simulink model "Red_problema7_imc_v2021"  (R2021a)
settings: Solver=ode15s  StartTime=0.0  StopTime=sim_time  RelTol=1e-3
values from neighbouring files (symbols this model uses):
  aE1 = a121_f    (= 50.6984417257)    [inicializar_areas_ej7.m]
  aE2 = a112_f    (= 77.7288481128)    [inicializar_areas_ej7.m]
  aE3 = a222_f    (= 163.424628674)    [inicializar_areas_ej7.m]
  aE4 = a213_f    (= 304.960661681)    [inicializar_areas_ej7.m]
  aEcu1 = aEcu1_f    (= 4.92677788377)    [inicializar_areas_ej7.m]
  aEcu2 = aEcu2_f    (= 18.7854640224)    [inicializar_areas_ej7.m]
  aEhu2 = aEhu2_f    (= 81.1441370104)    [inicializar_areas_ej7.m]
  d1_end = 0    [script_build_tfs.m]    (also in todo_nom_full.m; todo_nom_spar.m)
  d1_in = 0    [script_build_tfs.m]    (also in todo_nom_full.m; todo_nom_spar.m)
  d2_end = 0    [script_build_tfs.m]    (also in todo_nom_full.m; todo_nom_spar.m)
  d2_in = 0    [script_build_tfs.m]    (also in todo_nom_full.m; todo_nom_spar.m)
  d3_end = 0    [script_build_tfs.m]    (also in todo_nom_full.m; todo_nom_spar.m)
  d3_in = 0    [script_build_tfs.m]    (also in todo_nom_full.m; todo_nom_spar.m)
  d4_end = 0    [script_build_tfs.m]    (also in todo_nom_full.m; todo_nom_spar.m)
  d4_in = 0    [script_build_tfs.m]    (also in todo_nom_full.m; todo_nom_spar.m)
  d5_end = 0    [script_build_tfs.m]    (also in todo_nom_full.m; todo_nom_spar.m)
  d5_in = 0    [script_build_tfs.m]    (also in todo_nom_full.m; todo_nom_spar.m)
  d6_end = 0    [script_build_tfs.m]    (also in todo_nom_full.m; todo_nom_spar.m)
  d6_in = 0    [script_build_tfs.m]    (also in todo_nom_full.m; todo_nom_spar.m)
  d7_end = 0    [script_build_tfs.m]    (also in todo_nom_full.m; todo_nom_spar.m)
  d7_in = 0    [script_build_tfs.m]    (also in todo_nom_full.m; todo_nom_spar.m)
  d8_end = 0    [script_build_tfs.m]    (also in todo_nom_full.m; todo_nom_spar.m)
  d8_in = 0    [script_build_tfs.m]    (also in todo_nom_full.m; todo_nom_spar.m)
  fcu2 = 5    [ini_comun.m]    (also in inicializar_areas_ej7.m; script_build_tfs.m; script_ini_ej7.m)
  fhu2 = 15    [ini_comun.m]    (also in inicializar_areas_ej7.m; script_build_tfs.m; script_ini_ej7.m)
  hcu = 1    [ini_comun.m]    (also in script_build_tfs.m; script_ini_ej7.m)
  hhu = 1    [ini_comun.m]    (also in script_build_tfs.m; script_ini_ej7.m)
  initials = nominales_u_full    [script_build_tfs.m]    (also in script_desc.m = nominales_u_desc; script_full.m; script_ini_ej7.m; script_spar.m = nominales_u_spar)
  s1 = 30    [ini_comun.m]    (also in script_build_tfs.m; script_ini_ej7.m)
  salida_pto_op = [432.98548652 333.041991092 482.910853128 483.037830645]    [D_desc_v1.mat]    (also in D_full_v1.mat = [432.959604691 333.033592475 482.878829311 483.126301479]; D_spar_v1.mat = [433.148784168 333.052277913 483.093095371 482.96198908]; salida_pt_op_desc.mat = [432.94450339 332.966292174 482.988443985 483.057252903]; salida_pt_op_desc_v2021.mat)
  setpoints = [160+273 60+273 210+273 210+273]    [ini_comun.m]    (also in script_build_tfs.m; script_ini_ej7.m)
  switch_var = 2    [script_IMC_ej7.m]    (also in script_desc.m = 0; script_full.m; script_spar.m = 1)
  t_step = 2000    [ini_comun.m]    (also in script_build_tfs.m = 300; script_ini_ej7.m = 600; validacion.m = 500)
  Tcuin = 288    [ini_comun.m]    (also in script_build_tfs.m; script_ini_ej7.m)
  Thuin = 523    [ini_comun.m]    (also in script_build_tfs.m; script_ini_ej7.m)
libraries: simulink x5, cstblocks x2
(part 1 of 2)
settings Model: Creator=Lautaro  LastModifiedBy=fzpat
settings SolverCC: AlgebraicLoopSolver=TrustRegion
settings DataIOCC: LimitDataPoints=on  SaveFormat=Array  ReturnWorkspaceOutputs=off
settings OptimizationCC: BlockReduction=off  BooleanDataType=off  LifeSpan=inf
settings DebuggingCC: SaveWithParameterizedLinksMsg=none  UnderspecifiedInitializationDetection=Classic  MergeDetectMultiDrivingBlocksExec=none  SignalResolutionControl=TryResolveAllWithWarning  SFUnexpectedBacktrackingDiag=warning  SFNoUnconditionalDefaultTransitionDiag=warning  SFExecutionAtInitializationDiag=none  ArithmeticOperatorsInVariantConditions=warning
settings HardwareCC: ProdBitPerPointer=32  ProdBitPerSizeT=32  ProdBitPerPtrDiffT=32  ProdLargestAtomicFloat=None  ProdIntDivRoundTo=Undefined  ProdEndianess=Unspecified  ProdWordSize=32  ProdHWDeviceType=32-bit Generic  TargetUnknown=on
settings ModelReferenceCC: PropagateSignalLabelsOutOfModel=off
settings SFSimCC: SimUseLocalCustomCode=off  CustomCodeUndefinedFunction=UseInterfaceOnly
settings RTWCC: RTWUseLocalCustomCode=off
settings CodeAppCC: StateflowObjectComments=on
settings GRTTargetCC: TargetLangStandard=C89/C90 (ANSI)
settings ConfigComp: CovMetricSettings=dw  CovSaveCumulativeToWorkspaceVar=on  CovSaveSingleToWorkspaceVar=on  CovExternalEMLEnable=off  CovSFcnEnable=off

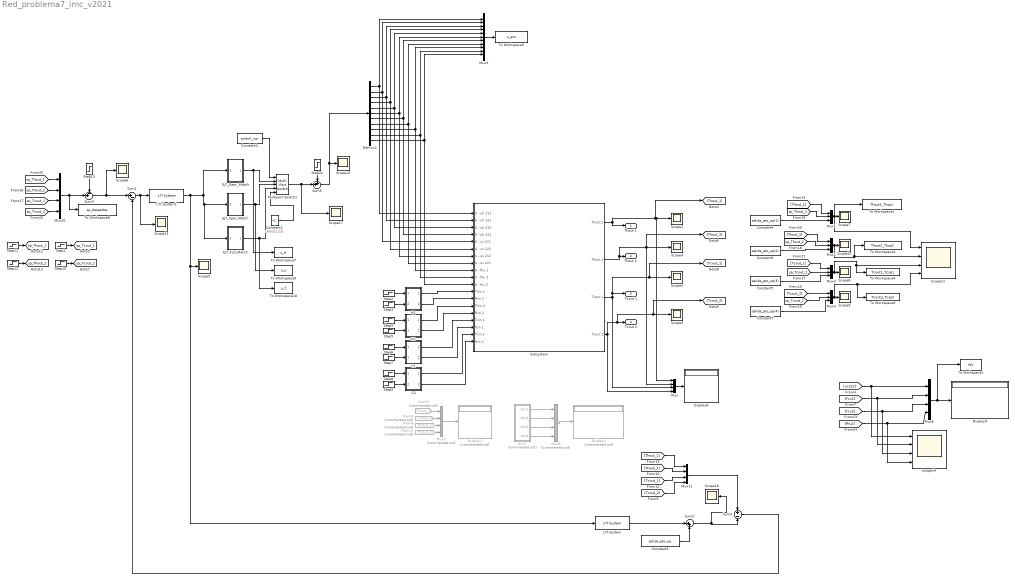
== system Red_problema7_imc_v2021 ==
  C1 : Subsystem
  "C2 " : Subsystem
  Constant1 : Constant  Value=zeros(1,11)
  Constant2 : Constant  Value=switch_var
  Constant3 : Constant  Value=salida_pto_op
  Constant4 : Constant  Value=salida_pto_op(1)
  Constant5 : Constant  Value=salida_pto_op(3)
  Constant6 : Constant  Value=salida_pto_op(2)
  Constant7 : Constant  Value=salida_pto_op(4)
  Demux2 : Demux  Outputs=11
  Display1 : Display  Commented=on
  Display5 : Display  Commented=on
  Display8 : Display
  Display9 : Display
  Ej7_Desc_Match : Subsystem
  Ej7_Full_Match : Subsystem
  Ej7_Spar_Match : Subsystem
  From11 : From  Commented=on  GotoTag=Tcout_2  TagVisibility=global
  From5 : From  Commented=on  GotoTag=Thout_1  TagVisibility=global
  From6 : From  Commented=on  GotoTag=Thout_2  TagVisibility=global
  From8 : From  Commented=on  GotoTag=Tcout_1  TagVisibility=global
  "H1 " : Subsystem
  H2 : Subsystem
  LTI System : cstblocks/LTI System  sys=Gimc  IC=[]
  LTI System1 : cstblocks/LTI System  sys=Kimc_u  IC=[]
  Multiport Switch1 : MultiPortSwitch  DataPortOrder=Zero-based contiguous  DataPortForDefault=Additional data port  DiagnosticForDefault=None  zeroidx=on
  Mux{,6,10..11} (4 alike) : Mux
  Mux{1..4} (4 alike) : Mux  Inputs=3
  Mux5 : Mux  Inputs=11
  Mux7 : Mux  Commented=on
  Mux8 : Mux  Commented=on
  Scope{1..10,12..13,17..18} (14 alike) : Scope
  Scope11 : Scope  NumInputPorts=4
  Scope14 : Scope  NumInputPorts=4
  Step1 : Step  Time=1e9  Before=210+273  After=210+273
  Step10 : Step  Time=1e10  Before=210+273  After=210+273
  Step11 : Step  Time=1e9  Before=160+273  After=160+273
  Step12 : Step  Time=1e9  Before=60+273  After=60+273
  Step13 : Step  Time=0  Before=setpoints  After=salida_pto_op
  Step2 : Step  Time=t_step  Before=d1_in  After=d1_end
  Step22 : Step  Time=0  Before=initials  After=initials
  Step3 : Step  Time=t_step  Before=d2_in  After=d2_end
  Step4 : Step  Time=t_step  Before=d3_in  After=d3_end
  Step5 : Step  Time=t_step  Before=d4_in  After=d4_end
  Step6 : Step  Time=t_step  Before=d5_in  After=d5_end
  Step7 : Step  Time=t_step  Before=d6_in  After=d6_end
  Step8 : Step  Time=t_step  Before=d7_in  After=d7_end
  Step9 : Step  Time=t_step  Before=d8_in  After=d8_end
  Subsystem : Subsystem
  Sum1 : Sum  Inputs=|+-
  Sum2 : Sum  Inputs=|++
  Sum3 : Sum  Inputs=+-
  Sum4 : Sum  Inputs=-+|
  Sum5 : Sum  Inputs=++|
  To Workspace1 : ToWorkspace  VariableName=MV  SaveFormat=Timeseries  SampleTime=-1
  To Workspace10 : ToWorkspace  VariableName=u_f  SaveFormat=Timeseries  SampleTime=-1
      settings: Save2DSignal=2-D array (concatenate along first dimension)
  To Workspace2 : ToWorkspace  VariableName=Thout1_Thsp1  SaveFormat=Timeseries  SampleTime=-1
  To Workspace3 : ToWorkspace  VariableName=Thout2_Thsp2  SampleTime=-1
  To Workspace4 : ToWorkspace  VariableName=Tcout1_Tcsp1  SampleTime=-1
  To Workspace5 : ToWorkspace  VariableName=u_exc  SaveFormat=Timeseries  SampleTime=-1
      settings: Save2DSignal=2-D array (concatenate along first dimension)
  To Workspace6 : ToWorkspace  VariableName=Tcout2_Tcsp2  SampleTime=-1
  To Workspace7 : ToWorkspace  VariableName=u_d  SaveFormat=Timeseries  SampleTime=-1
      settings: Save2DSignal=2-D array (concatenate along first dimension)
  To Workspace8 : ToWorkspace  VariableName=sp_deseados  SampleTime=-1
  To Workspace9 : ToWorkspace  VariableName=u_s  SaveFormat=Timeseries  SampleTime=-1
      settings: Save2DSignal=2-D array (concatenate along first dimension)
  error : Subsystem  Commented=on
  Thout 1 : Outport  VectorParamsAs1DForOutWhenUnconnected=off
  Thout 2 : Outport  Port=2  VectorParamsAs1DForOutWhenUnconnected=off
  Tcout 1 : Outport  Port=3  VectorParamsAs1DForOutWhenUnconnected=off
  Tcout 2 : Outport  Port=4  VectorParamsAs1DForOutWhenUnconnected=off
  tag scope: sp_Tcout_1=global, sp_Tcout_2=global, sp_Thout_1=global, sp_Thout_2=global
  wires:
  Subsystem/1(Thout 1) -> Thout 1/1, [Thout_1], Mux/1, Scope1/1
  Mux/1 -> Display8/1
  "H1 "/1(Out1) -> Subsystem/12(Thin 1)
  "H1 "/2(Out2) -> Subsystem/13(fhin 1)
  H2/2(Out2) -> Subsystem/15(fhin 2)
  H2/1(Out1) -> Subsystem/14(Thin 2)
  C1/1(Out1) -> Subsystem/16(Tcin 1)
  C1/2(Out2) -> Subsystem/17(fcin 1)
  "C2 "/1(Out1) -> Subsystem/18(Tcin 2)
  "C2 "/2(Out2) -> Subsystem/19(fcin 2)
  Subsystem/2(Thout 2) -> [Thout_2], Scope4/1, Mux/2, Thout 2/1
  Subsystem/3(Tcout 1) -> [Tcout_1], Scope2/1, Tcout 1/1, Mux/3
  Step2/1 -> "H1 "/1(Thin 1)
  Step3/1 -> "H1 "/2(fhin 1)
  Step4/1 -> H2/1(Thin 1)
  Step5/1 -> H2/2(fhin 1)
  Step6/1 -> C1/1(Tcin 1)
  Step7/1 -> C1/2(fcin 1)
  Step8/1 -> "C2 "/1(Tcin 2)
  Step9/1 -> "C2 "/2(fcin 2)
  Subsystem/4(Tcout 2) -> [Tcout_2], Scope3/1, Tcout 2/1, Mux/4
  Mux5/1 -> To Workspace5/1
  Mux7/1 -> Display1/1
  From6/1 -> Mux7/2
  error/3(Out3) -> Mux8/3
  From5/1 -> Mux7/1
  From11/1 -> Mux7/4
  From8/1 -> Mux7/3
  error/4(Out4) -> Mux8/4
  Mux8/1 -> Display5/1
  Step12/1 -> [sp_Thout_2]
  Step11/1 -> [sp_Thout_1]
  Step1/1 -> [sp_Tcout_1]
  Step10/1 -> [sp_Tcout_2]
  error/2(Out2) -> Mux8/2
  error/1(Out1) -> Mux8/1
  [Tcout_1] -> Mux3/1
  Mux3/1 -> To Workspace4/1, Scope11/3, Scope8/1
  [Thout_2] -> Mux2/1
  [sp_Tcout_1] -> Mux3/2
  Mux1/1 -> To Workspace2/1, Scope11/1, Scope7/1
  Mux2/1 -> To Workspace3/1, Scope11/2, Scope10/1
  [Tcout_2] -> Mux4/1
  [Thout_1] -> Mux1/1
  Mux4/1 -> To Workspace6/1, Scope11/4, Scope9/1
  [sp_Thout_2] -> Mux2/2
  [sp_Tcout_2] -> Mux4/2
  [sp_Thout_1] -> Mux1/2
  [fcu1] -> Mux6/2, Scope14/2
  [fhu2] -> Scope14/4, Mux6/4
  [uc222] -> Mux6/1, Scope14/1
  [fcu2] -> Mux6/3, Scope14/3
  Mux6/1 -> To Workspace1/1, Display9/1
  [sp_Tcout_1] -> Mux10/3
  [sp_Thout_2] -> Mux10/2
  [sp_Thout_1] -> Mux10/1
  Sum2/1 -> Sum3/2, Scope18/1
  [sp_Tcout_2] -> Mux10/4
  Mux10/1 -> To Workspace8/1, Sum4/2
  Sum1/1 -> Scope13/1, LTI System1/1
  Ej7_Spar_Match/1(Out1) -> To Workspace9/1, Multiport Switch1/3
  Constant1/1 -> Multiport Switch1/5
  Ej7_Full_Match/1(Out1) -> To Workspace10/1, Multiport Switch1/4
  Ej7_Desc_Match/1(Out1) -> Multiport Switch1/2, To Workspace7/1
  Constant2/1 -> Multiport Switch1/1
  Mux11/1 -> Sum3/1
  [Thout_2] -> Mux11/2
  Constant3/1 -> Sum2/2
  [Tcout_1] -> Mux11/3
  [Thout_1] -> Mux11/1
  LTI System/1 -> Sum2/1
  [Tcout_2] -> Mux11/4
  Demux2/10 -> Subsystem/10(U - fhu 2), Mux5/10
  Step22/1 -> Sum5/1
  Demux2/4 -> Mux5/4, Subsystem/6(U - uc 121)
  Demux2/3 -> Mux5/3, Subsystem/2(U - uh 121)
  Demux2/7 -> Mux5/7, Subsystem/4(U - uh 221)
  Demux2/8 -> Mux5/8, Subsystem/8(U - uc 221)
  Demux2/11 -> Mux5/11, Subsystem/11(U - fcu 2)
  Demux2/5 -> Mux5/5, Subsystem/3(U - uh 212)
  Demux2/9 -> Subsystem/9(U - fhu 1), Mux5/9
  Demux2/6 -> Mux5/6, Subsystem/7(U - uc 212)
  Demux2/1 -> Mux5/1, Subsystem/1(U - uh 111)
  Demux2/2 -> Mux5/2, Subsystem/5(U - uc 111)
  Multiport Switch1/1 -> Scope17/1, Sum5/2
  Sum3/1 -> Sum1/2
  Sum4/1 -> Scope6/1, Sum1/1
  Step13/1 -> Sum4/1
  Sum5/1 -> Demux2/1, Scope12/1
  LTI System1/1 -> LTI System/1, Scope5/1, Ej7_Desc_Match/1(In1), Ej7_Full_Match/1(In1), Ej7_Spar_Match/1(In1)
  Constant4/1 -> Mux1/3
  Constant6/1 -> Mux2/3
  Constant5/1 -> Mux3/3
  Constant7/1 -> Mux4/3

== system Red_problema7_imc_v2021/C1 ==
  Tcin 1 : Inport
  fcin 1 : Inport  Port=2
  Add2 : Sum
  Add3 : Sum
  Constant3 : Constant  Value=50+273
  Constant4 : Constant  Value=20
  Out1 : Outport  VectorParamsAs1DForOutWhenUnconnected=off
  Out2 : Outport  Port=2  VectorParamsAs1DForOutWhenUnconnected=off
  wires:
  Constant3/1 -> Add2/1
  Constant4/1 -> Add3/1
  Tcin 1/1 -> Add2/2
  fcin 1/1 -> Add3/2
  Add2/1 -> Out1/1
  Add3/1 -> Out2/1

== system Red_problema7_imc_v2021/C2  ==
  Tcin 2 : Inport
  fcin 2 : Inport  Port=2
  Add4 : Sum
  Add5 : Sum
  Constant5 : Constant  Value=160+273
  Constant6 : Constant  Value=50
  Out1 : Outport  VectorParamsAs1DForOutWhenUnconnected=off
  Out2 : Outport  Port=2  VectorParamsAs1DForOutWhenUnconnected=off
  wires:
  Constant5/1 -> Add4/1
  Constant6/1 -> Add5/1
  Tcin 2/1 -> Add4/2
  fcin 2/1 -> Add5/2
  Add4/1 -> Out1/1
  Add5/1 -> Out2/1

== system Red_problema7_imc_v2021/Ej7_Desc_Match ==
  In1 : Inport
  Constant1 : Constant  Value=0
  Demux3 : Demux
  Mux10 : Mux  Inputs=11
  Out1 : Outport
  wires:
  In1/1 -> Demux3/1
  Constant1/1 -> Mux10/3, Mux10/5, Mux10/7, Mux10/6, Mux10/4, Mux10/2, Mux10/1
  Demux3/4 -> Mux10/11
  Demux3/2 -> Mux10/10
  Demux3/1 -> Mux10/9
  Mux10/1 -> Out1/1
  Demux3/3 -> Mux10/8

== system Red_problema7_imc_v2021/Ej7_Full_Match ==
  In1 : Inport
  Constant1 : Constant  Value=0
  Constant2 : Constant  Value=0
  Constant3 : Constant  Value=0
  Demux3 : Demux
  Mux10 : Mux  Inputs=11
  Out1 : Outport
  wires:
  Constant3/1 -> Mux10/11
  In1/1 -> Demux3/1
  Constant2/1 -> Mux10/7, Mux10/4, Mux10/3, Mux10/5, Mux10/6
  Constant1/1 -> Mux10/1
  Demux3/4 -> Mux10/8
  Demux3/3 -> Mux10/2
  Demux3/2 -> Mux10/10
  Demux3/1 -> Mux10/9
  Mux10/1 -> Out1/1

== system Red_problema7_imc_v2021/Ej7_Spar_Match ==
  In1 : Inport
  Constant1 : Constant  Value=0
  Constant2 : Constant  Value=0
  Demux3 : Demux
  Mux10 : Mux  Inputs=11
  Out1 : Outport
  wires:
  Mux10/1 -> Out1/1
  Demux3/1 -> Mux10/9
  Demux3/2 -> Mux10/10
  Demux3/3 -> Mux10/5
  Demux3/4 -> Mux10/11
  Constant1/1 -> Mux10/4, Mux10/3, Mux10/2, Mux10/1
  Constant2/1 -> Mux10/6, Mux10/8, Mux10/7
  In1/1 -> Demux3/1

== system Red_problema7_imc_v2021/H1  ==
  Thin 1 : Inport
  fhin 1 : Inport  Port=2
  Add : Sum
  Add1 : Sum
  Constant1 : Constant  Value=270+273
  Constant2 : Constant  Value=18
  Out1 : Outport  VectorParamsAs1DForOutWhenUnconnected=off
  Out2 : Outport  Port=2  VectorParamsAs1DForOutWhenUnconnected=off
  wires:
  Constant1/1 -> Add/1
  Thin 1/1 -> Add/2
  Add/1 -> Out1/1
  Constant2/1 -> Add1/1
  fhin 1/1 -> Add1/2
  Add1/1 -> Out2/1

== system Red_problema7_imc_v2021/H2 ==
  Thin 1 : Inport
  fhin 1 : Inport  Port=2
  Add : Sum
  Add1 : Sum
  Constant1 : Constant  Value=220+273
  Constant2 : Constant  Value=22
  Out1 : Outport  VectorParamsAs1DForOutWhenUnconnected=off
  Out2 : Outport  Port=2  VectorParamsAs1DForOutWhenUnconnected=off
  wires:
  Constant1/1 -> Add/1
  Thin 1/1 -> Add/2
  Add/1 -> Out1/1
  Constant2/1 -> Add1/1
  fhin 1/1 -> Add1/2
  Add1/1 -> Out2/1

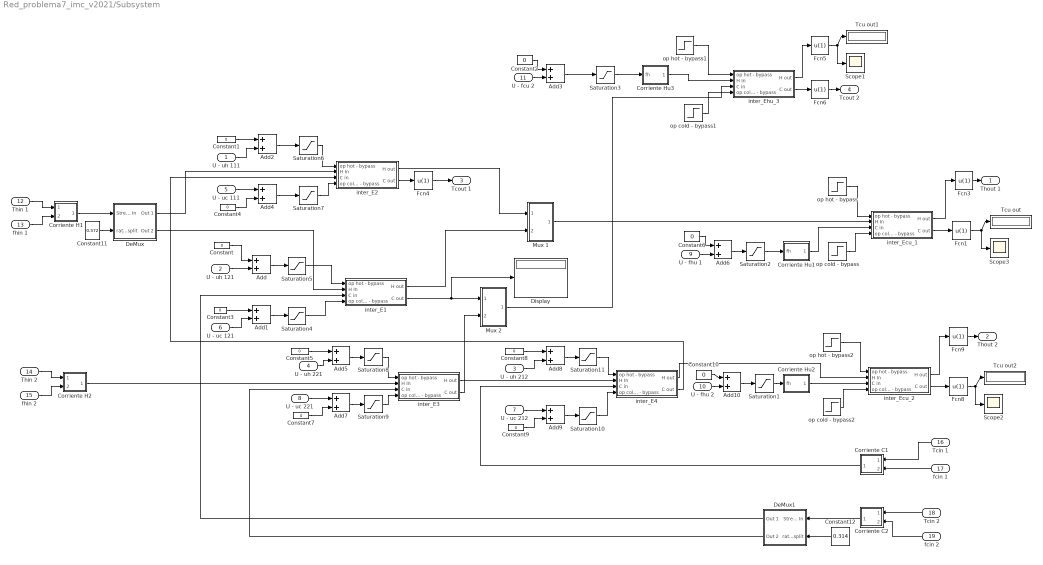
== system Red_problema7_imc_v2021/Subsystem ==
  U - uh 111 : Inport
  U - uh 121 : Inport  Port=2
  U - uh 212 : Inport  Port=3
  U - uh 221 : Inport  Port=4
  U - uc 111 : Inport  Port=5
  U - uc 121 : Inport  Port=6
  U - uc 212 : Inport  Port=7
  U - uc 221 : Inport  Port=8
  U - fhu 1 : Inport  Port=9
  U - fhu 2 : Inport  Port=10
  U - fcu 2 : Inport  Port=11
  Thin 1 : Inport  Port=12
  fhin 1 : Inport  Port=13
  Thin 2 : Inport  Port=14
  fhin 2 : Inport  Port=15
  Tcin 1 : Inport  Port=16
  fcin 1 : Inport  Port=17
  Tcin 2 : Inport  Port=18
  fcin 2 : Inport  Port=19
  Add{,1..10} (11 alike) : Sum
  Constant{,1..10} (11 alike) : Constant  Value=0
  Constant11 : Constant  Value=0.572
  Constant12 : Constant  Value=0.314
  Corriente C1 : Subsystem
  Corriente C2 : Subsystem
  Corriente H1 : Subsystem
  Corriente H2 : Subsystem
  Corriente Hu1 : Subsystem
  Corriente Hu2 : Subsystem
  Corriente Hu3 : Subsystem
  DeMux : Subsystem
  DeMux1 : Subsystem
  Display : Display
  Fcn{1,3..6,8..9} (7 alike) : Fcn  Expr=u(1)
  "Mux 1 " : Subsystem
  Mux 2 : Subsystem
  Saturation1 : Saturate  UpperLimit=1e9  LowerLimit=0
  Saturation{4..11} (8 alike) : Saturate  UpperLimit=1e9  LowerLimit=1e-3
  Saturation2 : Saturate  UpperLimit=1e9  LowerLimit=0
  Saturation3 : Saturate  UpperLimit=1e9  LowerLimit=0
  Scope1 : Scope
  Scope2 : Scope
  Scope3 : Scope
  Tcu out : Display
  Tcu out1 : Display
  Tcu out2 : Display
  inter_E1 : Subsystem
  inter_E2 : Subsystem
  inter_E3 : Subsystem
  inter_E4 : Subsystem
  inter_Ecu_1 : Subsystem
  inter_Ecu_2 : Subsystem
  inter_Ehu_3 : Subsystem
  op cold - bypass : Step  Time=0  After=0  SampleTime=0
  op cold - bypass1 : Step  Time=0  After=0  SampleTime=0
  op cold - bypass2 : Step  Time=0  After=0  SampleTime=0
  op hot - bypass : Step  Time=0  After=0  SampleTime=0
  op hot - bypass1 : Step  Time=0  After=0  SampleTime=0
  op hot - bypass2 : Step  Time=0  After=0  SampleTime=0
  Thout 1 : Outport  VectorParamsAs1DForOutWhenUnconnected=off
  Thout 2 : Outport  Port=2  VectorParamsAs1DForOutWhenUnconnected=off
  Tcout 1 : Outport  Port=3  VectorParamsAs1DForOutWhenUnconnected=off
  Tcout 2 : Outport  Port=4  VectorParamsAs1DForOutWhenUnconnected=off
  wires:
  op cold - bypass/1 -> inter_Ecu_1/4("op cold - bypass ")
  Fcn1/1 -> Scope3/1, Tcu out/1
  op hot - bypass/1 -> inter_Ecu_1/1("op hot - bypass ")
  Thin 1/1 -> Corriente H1/1(In1)
  fhin 1/1 -> Corriente H1/2(In2)
  Tcin 1/1 -> Corriente C1/1(In1)
  fcin 1/1 -> Corriente C1/2(In2)
  Tcin 2/1 -> Corriente C2/1(In1)
  fcin 2/1 -> Corriente C2/2(In2)
  U - uh 121/1 -> Add/2
  Constant/1 -> Add/1
  U - uc 121/1 -> Add1/2
  Add1/1 -> Saturation4/1
  Add/1 -> Saturation5/1
  U - uh 111/1 -> Add2/2
  Constant1/1 -> Add2/1
  Add2/1 -> Saturation6/1
  Constant3/1 -> Add1/1
  U - uc 111/1 -> Add4/1
  Constant4/1 -> Add4/2
  Add4/1 -> Saturation7/1
  Add6/1 -> Saturation2/1
  U - fhu 1/1 -> Add6/2
  Constant6/1 -> Add6/1
  Thin 2/1 -> Corriente H2/1(In1)
  fhin 2/1 -> Corriente H2/2(In2)
  op cold - bypass1/1 -> inter_Ehu_3/4("op cold - bypass ")
  Fcn5/1 -> Scope1/1, Tcu out1/1
  op hot - bypass1/1 -> inter_Ehu_3/1("op hot - bypass ")
  Add3/1 -> Saturation3/1
  U - fcu 2/1 -> Add3/2
  Constant2/1 -> Add3/1
  Corriente Hu3/1(Out1) -> inter_Ehu_3/2(H In)
  inter_Ehu_3/2(C out) -> Fcn6/1
  inter_Ehu_3/1(H out) -> Fcn5/1
  Fcn4/1 -> Tcout 1/1
  Fcn6/1 -> Tcout 2/1
  Fcn3/1 -> Thout 1/1
  Corriente Hu1/1(Out1) -> inter_Ecu_1/3(C in)
  inter_Ecu_1/2(C out) -> Fcn1/1
  inter_Ecu_1/1(H out) -> Fcn3/1
  U - uh 221/1 -> Add5/2
  Constant5/1 -> Add5/1
  Add5/1 -> Saturation8/1
  U - uc 221/1 -> Add7/1
  Constant7/1 -> Add7/2
  Add7/1 -> Saturation9/1
  U - uh 212/1 -> Add8/2
  Constant8/1 -> Add8/1
  Add8/1 -> Saturation11/1
  U - uc 212/1 -> Add9/1
  Constant9/1 -> Add9/2
  Add9/1 -> Saturation10/1
  op cold - bypass2/1 -> inter_Ecu_2/4("op cold - bypass ")
  Fcn8/1 -> Scope2/1, Tcu out2/1
  op hot - bypass2/1 -> inter_Ecu_2/1("op hot - bypass ")
  Add10/1 -> Saturation1/1
  U - fhu 2/1 -> Add10/2
  Constant10/1 -> Add10/1
  Fcn9/1 -> Thout 2/1
  Corriente Hu2/1(Out1) -> inter_Ecu_2/3(C in)
  inter_Ecu_2/2(C out) -> Fcn8/1
  inter_Ecu_2/1(H out) -> Fcn9/1
  inter_E2/2(C out) -> Fcn4/1
  Constant11/1 -> DeMux/2("ratio split ")
  Corriente H1/1(Out1) -> DeMux/1(Strem In)
  DeMux/2(Out 2) -> inter_E1/2(H In)
  DeMux/1(Out 1) -> inter_E2/2(H In)
  Constant12/1 -> DeMux1/2("ratio split ")
  Corriente C2/1(Out1) -> DeMux1/1(Strem In)
  DeMux1/1(Out 1) -> inter_E1/3(C in)
  Corriente H2/1(Out1) -> inter_E3/2(H In)
  inter_E3/1(H out) -> inter_E4/2(H In)
  inter_E2/1(H out) -> "Mux 1 "/1(in 1)
  inter_E1/1(H out) -> "Mux 1 "/2(in 2)
  "Mux 1 "/1(Out) -> inter_Ecu_1/2(H In)
  DeMux1/2(Out 2) -> inter_E3/3(C in)
  inter_E1/2(C out) -> Display/1, Mux 2/1(in 1)
  inter_E3/2(C out) -> Mux 2/2(in 2)
  inter_E4/1(H out) -> inter_Ecu_2/2(H In)
  Mux 2/1(Out) -> inter_Ehu_3/3(C in)
  Corriente C1/1(Out1) -> inter_E4/3(C in)
  inter_E4/2(C out) -> inter_E2/3(C in)
  Saturation1/1 -> Corriente Hu2/1(fh)
  Saturation2/1 -> Corriente Hu1/1(fh)
  Saturation3/1 -> Corriente Hu3/1(fh)
  Saturation4/1 -> inter_E1/4("op cold - bypass ")
  Saturation5/1 -> inter_E1/1("op hot - bypass ")
  Saturation6/1 -> inter_E2/1("op hot - bypass ")
  Saturation7/1 -> inter_E2/4("op cold - bypass ")
  Saturation8/1 -> inter_E3/1("op hot - bypass ")
  Saturation9/1 -> inter_E3/4("op cold - bypass ")
  Saturation10/1 -> inter_E4/4("op cold - bypass ")
  Saturation11/1 -> inter_E4/1("op hot - bypass ")

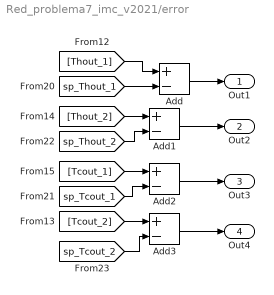
== system Red_problema7_imc_v2021/error ==
  Add{,1..3} (4 alike) : Sum  Inputs=+-
  Out1 : Outport  VectorParamsAs1DForOutWhenUnconnected=off
  Out2 : Outport  Port=2  VectorParamsAs1DForOutWhenUnconnected=off
  Out3 : Outport  Port=3  VectorParamsAs1DForOutWhenUnconnected=off
  Out4 : Outport  Port=4  VectorParamsAs1DForOutWhenUnconnected=off
  wires:
  [sp_Thout_2] -> Add1/2
  [sp_Tcout_2] -> Add3/2
  [sp_Tcout_1] -> Add2/2
  [sp_Thout_1] -> Add/2
  [Thout_2] -> Add1/1
  [Thout_1] -> Add/1
  [Tcout_1] -> Add2/1
  [Tcout_2] -> Add3/1
  Add1/1 -> Out2/1
  Add/1 -> Out1/1
  Add3/1 -> Out4/1
  Add2/1 -> Out3/1

== system Red_problema7_imc_v2021/Subsystem/Corriente C1 ==
  In1 : Inport
  In2 : Inport  Port=2
  Mux5 : Mux  Inputs=3
  Terminator : Terminator
  Terminator1 : Terminator
  fc : Step  Before=13  After=13  SampleTime=0
  hc : Step  Before=1  SampleTime=0
  tc : Step  Before=333  After=333  SampleTime=0
  valvula 3 : Subsystem
  Out1 : Outport  VectorParamsAs1DForOutWhenUnconnected=off
  wires:
  Mux5/1 -> valvula 3/1(In1)
  hc/1 -> Mux5/3
  In1/1 -> Mux5/1
  In2/1 -> Mux5/2
  fc/1 -> Terminator/1
  tc/1 -> Terminator1/1
  valvula 3/1(Out1) -> Out1/1

== system Red_problema7_imc_v2021/Subsystem/Corriente C2 ==
  In1 : Inport
  In2 : Inport  Port=2
  Mux5 : Mux  Inputs=3
  Terminator : Terminator
  Terminator1 : Terminator
  fh : Step  Before=12  After=12  SampleTime=0
  hh : Step  Before=1  SampleTime=0
  th : Step  Time=2  Before=293  After=293  SampleTime=0
  valvula 3 : Subsystem
  Out1 : Outport  VectorParamsAs1DForOutWhenUnconnected=off
  wires:
  hh/1 -> Mux5/3
  Mux5/1 -> valvula 3/1(In1)
  In1/1 -> Mux5/1
  In2/1 -> Mux5/2
  fh/1 -> Terminator/1
  th/1 -> Terminator1/1
  valvula 3/1(Out1) -> Out1/1

== system Red_problema7_imc_v2021/Subsystem/Corriente H1 ==
  In1 : Inport
  In2 : Inport  Port=2
  Mux5 : Mux  Inputs=3
  Terminator : Terminator
  Terminator1 : Terminator
  fh : Step  Before=20  After=20  SampleTime=0
  hh : Step  Before=1  SampleTime=0
  th : Step  Time=2  Before=423  After=423  SampleTime=0
  valvula 3 : Subsystem
  Out1 : Outport  VectorParamsAs1DForOutWhenUnconnected=off
  wires:
  Mux5/1 -> valvula 3/1(In1)
  hh/1 -> Mux5/3
  In1/1 -> Mux5/1
  In2/1 -> Mux5/2
  th/1 -> Terminator/1
  fh/1 -> Terminator1/1
  valvula 3/1(Out1) -> Out1/1

== system Red_problema7_imc_v2021/Subsystem/Corriente H2 ==
  In1 : Inport
  In2 : Inport  Port=2
  Mux5 : Mux  Inputs=3
  Terminator : Terminator
  Terminator1 : Terminator
  fh : Step  Before=20  After=20  SampleTime=0
  hh : Step  Before=1  SampleTime=0
  th : Step  Time=2  Before=423  After=423  SampleTime=0
  valvula 3 : Subsystem
  Out1 : Outport  VectorParamsAs1DForOutWhenUnconnected=off
  wires:
  Mux5/1 -> valvula 3/1(In1)
  hh/1 -> Mux5/3
  In1/1 -> Mux5/1
  In2/1 -> Mux5/2
  th/1 -> Terminator/1
  fh/1 -> Terminator1/1
  valvula 3/1(Out1) -> Out1/1

== system Red_problema7_imc_v2021/Subsystem/Corriente Hu1 ==
  fh : Inport
  Mux5 : Mux  Inputs=3
  hh : Step  Before=1  SampleTime=0
  th : Step  Time=2  Before=15+273  After=15+273  SampleTime=0
  valvula 3 : Subsystem
  Out1 : Outport  VectorParamsAs1DForOutWhenUnconnected=off
  wires:
  hh/1 -> Mux5/3
  th/1 -> Mux5/1
  Mux5/1 -> valvula 3/1(In1)
  fh/1 -> Mux5/2
  valvula 3/1(Out1) -> Out1/1

== system Red_problema7_imc_v2021/Subsystem/Corriente Hu2 ==
  fh : Inport
  Mux5 : Mux  Inputs=3
  hh : Step  Before=1  SampleTime=0
  th : Step  Time=2  Before=15+273  After=15+273  SampleTime=0
  valvula 3 : Subsystem
  Out1 : Outport  VectorParamsAs1DForOutWhenUnconnected=off
  wires:
  hh/1 -> Mux5/3
  th/1 -> Mux5/1
  Mux5/1 -> valvula 3/1(In1)
  fh/1 -> Mux5/2
  valvula 3/1(Out1) -> Out1/1

== system Red_problema7_imc_v2021/Subsystem/Corriente Hu3 ==
  fh : Inport
  Mux5 : Mux  Inputs=3
  hh : Step  Before=1  SampleTime=0
  th : Step  Time=2  Before=250+273  After=250+273  SampleTime=0
  valvula 3 : Subsystem
  Out1 : Outport  VectorParamsAs1DForOutWhenUnconnected=off
  wires:
  hh/1 -> Mux5/3
  th/1 -> Mux5/1
  Mux5/1 -> valvula 3/1(In1)
  fh/1 -> Mux5/2
  valvula 3/1(Out1) -> Out1/1

== system Red_problema7_imc_v2021/Subsystem/DeMux ==
  note: split ratio relacionado con la Stream 1
  Strem In : Inport
  "ratio split " : Inport  Port=2
  Add : Sum  Inputs=-+
  Constant : Constant
  Demux : Demux  Outputs=3
  Mux : Mux  Inputs=3
  Mux1 : Mux  Inputs=3
  Product1 : Product
  Product2 : Product
  Out 1 : Outport  VectorParamsAs1DForOutWhenUnconnected=off
  Out 2 : Outport  Port=2  VectorParamsAs1DForOutWhenUnconnected=off
  wires:
  Strem In/1 -> Demux/1
  Mux/1 -> Out 1/1
  Mux1/1 -> Out 2/1
  Demux/3 -> Mux/3, Mux1/3
  Demux/1 -> Mux1/1, Mux/1
  "ratio split "/1 -> Add/1, Product2/1
  Demux/2 -> Product1/1, Product2/2
  Product2/1 -> Mux/2
  Constant/1 -> Add/2
  Add/1 -> Product1/2
  Product1/1 -> Mux1/2

== system Red_problema7_imc_v2021/Subsystem/DeMux1 ==
  note: split ratio relacionado con la Stream 1
  Strem In : Inport
  "ratio split " : Inport  Port=2
  Add : Sum  Inputs=-+
  Constant : Constant
  Demux : Demux  Outputs=3
  Mux : Mux  Inputs=3
  Mux1 : Mux  Inputs=3
  Product1 : Product
  Product2 : Product
  Out 1 : Outport  VectorParamsAs1DForOutWhenUnconnected=off
  Out 2 : Outport  Port=2  VectorParamsAs1DForOutWhenUnconnected=off
  wires:
  Strem In/1 -> Demux/1
  Mux/1 -> Out 1/1
  Mux1/1 -> Out 2/1
  Demux/3 -> Mux/3, Mux1/3
  Demux/1 -> Mux1/1, Mux/1
  "ratio split "/1 -> Add/1, Product2/1
  Demux/2 -> Product1/1, Product2/2
  Product2/1 -> Mux/2
  Constant/1 -> Add/2
  Add/1 -> Product1/2
  Product1/1 -> Mux1/2

== system Red_problema7_imc_v2021/Subsystem/Mux 1  ==
  in 1 : Inport
  in 2 : Inport  Port=2
  Add3 : Sum
  Add5 : Sum
  Demux : Demux  Outputs=3
  Demux1 : Demux  Outputs=3
  Divide : Product  Inputs=/*
  Mux : Mux  Inputs=3
  Product : Product
  Product1 : Product
  Terminator1 : Terminator
  Out : Outport  VectorParamsAs1DForOutWhenUnconnected=off
  wires:
  Product/1 -> Add3/1
  Product1/1 -> Add3/2
  Demux/1 -> Product/1
  Demux1/2 -> Add5/2, Product1/2
  Demux1/1 -> Product1/1
  Demux/2 -> Add5/1, Product/2
  Add5/1 -> Mux/2, Divide/1
  Add3/1 -> Divide/2
  in 2/1 -> Demux1/1
  in 1/1 -> Demux/1
  Demux1/3 -> Terminator1/1
  Divide/1 -> Mux/1
  Demux/3 -> Mux/3
  Mux/1 -> Out/1

== system Red_problema7_imc_v2021/Subsystem/Mux 2 ==
  in 1 : Inport
  in 2 : Inport  Port=2
  Add3 : Sum
  Add5 : Sum
  Demux : Demux  Outputs=3
  Demux1 : Demux  Outputs=3
  Display : Display
  Display1 : Display
  Divide : Product  Inputs=/*
  Mux : Mux  Inputs=3
  Product : Product
  Product1 : Product
  Terminator1 : Terminator
  Out : Outport  VectorParamsAs1DForOutWhenUnconnected=off
  wires:
  Product/1 -> Add3/1
  Product1/1 -> Add3/2
  Demux/1 -> Product/1
  Demux1/2 -> Display1/1, Add5/2, Product1/2
  Demux1/1 -> Product1/1
  Demux/2 -> Display/1, Add5/1, Product/2
  Add5/1 -> Mux/2, Divide/1
  Add3/1 -> Divide/2
  in 2/1 -> Demux1/1
  in 1/1 -> Demux/1
  Demux1/3 -> Terminator1/1
  Divide/1 -> Mux/1
  Demux/3 -> Mux/3
  Mux/1 -> Out/1

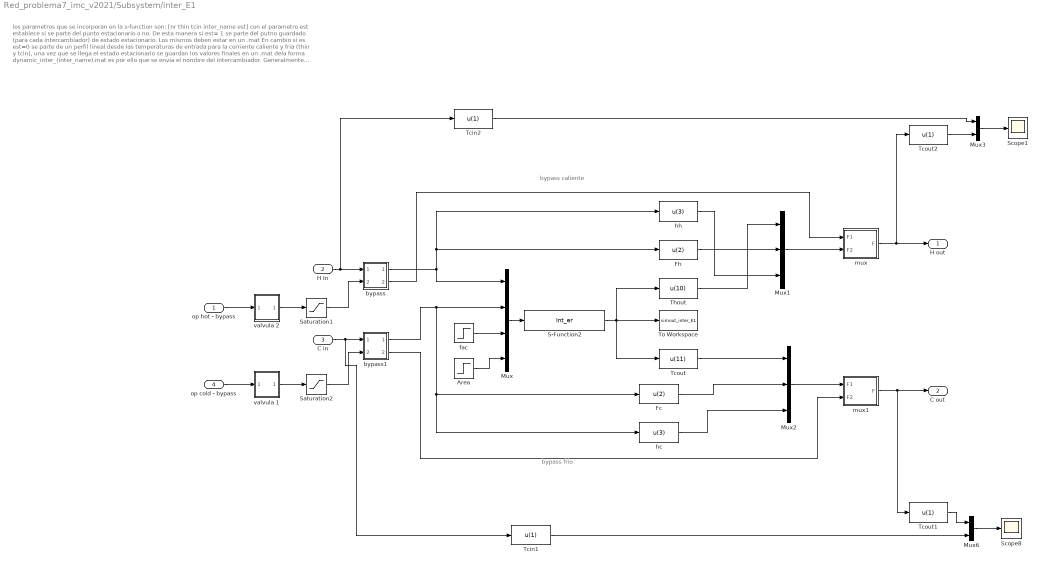
== system Red_problema7_imc_v2021/Subsystem/inter_E1 ==
  note: los parametros que se incorporan en la s-function son: [nr thin tcin inter_name est]
      | con el parametro est establece si se parte del punto estacionario o no. De esta manera si est= 1 se parte del putno guardado (para cada intercambiador) de estado estacionario. Los mismos deben estar en un .mat
      | En cambio si es est=0 se parte de un perfil lineal  desde las temperaturas de entrada para la corriente caliente y fria (thin y tcin), una vez que se llega el estado estacionario se guardan los valores finales en un .mat
      | dela forma dynamic_inter_(inter_name).mat   es por ello que se envia el nombre del intercambiador.
      | Generalmente para la primera vez que se corre la red se una est=0 para que llegue al estado estacionario y una vez que se alcanzó se vuelve a correr con est= 1 para hacer análisis de control
  note: bypass frio
  note: bypass caliente
  "op hot - bypass " : Inport
  H In : Inport  Port=2
  C in : Inport  Port=3
  "op cold - bypass " : Inport  Port=4
  Area : Step  Time=8  Before=aE1  After=aE1  SampleTime=0
  Fc : Fcn  Expr=u(2)
  Fh : Fcn  Expr=u(2)
  Mux : Mux
  Mux1 : Mux  Inputs=3
  Mux2 : Mux  Inputs=3
  Mux3 : Mux  Inputs=2
  Mux6 : Mux  Inputs=2
  S-Function2 : S-Function  FunctionName=Int_er  Parameters=10 543 433 121 2  SFunctionDeploymentMode=off  EnableBusSupport=off
  Saturation1 : Saturate  UpperLimit=1  LowerLimit=0
  Saturation2 : Saturate  UpperLimit=1  LowerLimit=0
  Scope1 : Scope
  Scope8 : Scope
  Tcin1 : Fcn  Expr=u(1)
  Tcin2 : Fcn  Expr=u(1)
  Tcout : Fcn  Expr=u(11)
  Tcout1 : Fcn  Expr=u(1)
  Tcout2 : Fcn  Expr=u(1)
  Thout : Fcn  Expr=u(10)
  To Workspace : ToWorkspace  VariableName=simout_inter_E1  SampleTime=-1
  bypass : Subsystem
  bypass1 : Subsystem
  fac : Step  After=0  SampleTime=0
  hc : Fcn  Expr=u(3)
  hh : Fcn  Expr=u(3)
  mux : Subsystem
  mux1 : Subsystem
  valvula 1 : Subsystem
  valvula 2 : Subsystem
  H out : Outport  VectorParamsAs1DForOutWhenUnconnected=off
  C out : Outport  Port=2  VectorParamsAs1DForOutWhenUnconnected=off
  wires:
  Tcout/1 -> Mux2/1
  Thout/1 -> Mux1/1
  Fc/1 -> Mux2/2
  Fh/1 -> Mux1/2
  S-Function2/1 -> Thout/1, To Workspace/1, Tcout/1
  Mux/1 -> S-Function2/1
  fac/1 -> Mux/3
  hc/1 -> Mux2/3
  hh/1 -> Mux1/3
  Area/1 -> Mux/4
  H In/1 -> Tcin2/1, bypass/1(1)
  bypass/1(" 1") -> Mux/1, Fh/1, hh/1
  Mux1/1 -> mux/2(F2)
  "op hot - bypass "/1 -> valvula 2/1(In1)
  C in/1 -> Tcin1/1, bypass1/1(1)
  "op cold - bypass "/1 -> valvula 1/1(In1)
  mux/1("F ") -> Tcout2/1, H out/1
  Mux2/1 -> mux1/1(F1)
  mux1/1("F ") -> Tcout1/1, C out/1
  bypass1/1(" 1") -> hc/1, Fc/1, Mux/2
  Mux6/1 -> Scope8/1
  Tcout1/1 -> Mux6/1
  Tcin1/1 -> Mux6/2
  Mux3/1 -> Scope1/1
  Tcout2/1 -> Mux3/2
  Tcin2/1 -> Mux3/1
  Saturation1/1 -> bypass/2(u122)
  Saturation2/1 -> bypass1/2(u122)
  bypass/2(" 2") -> mux/1(F1)
  bypass1/2(" 2") -> mux1/2(F2)
  valvula 1/1(Out1) -> Saturation2/1
  valvula 2/1(Out1) -> Saturation1/1

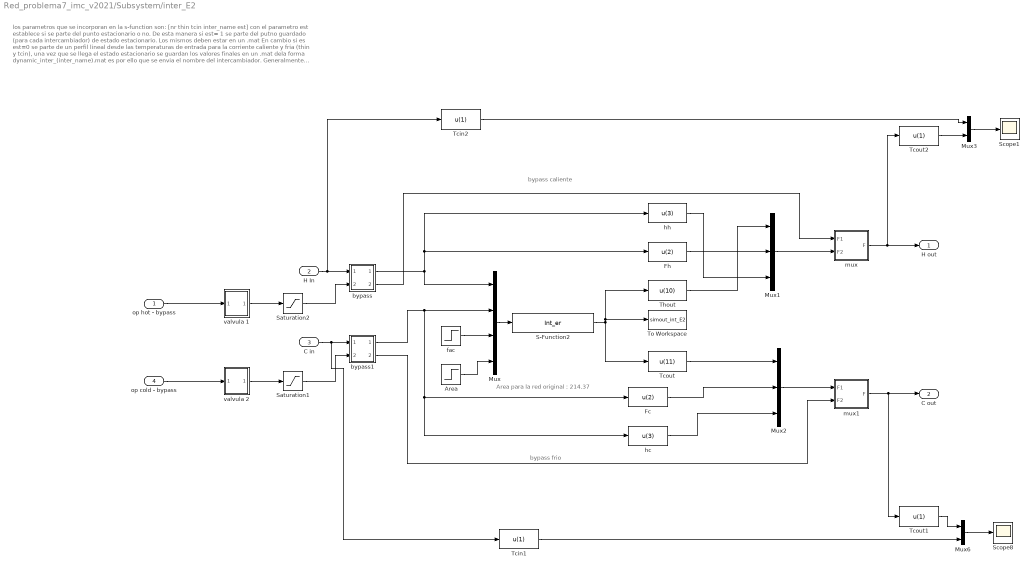
== system Red_problema7_imc_v2021/Subsystem/inter_E2 ==
  note: Area para la red original : 214.37
  note: bypass caliente
  note: bypass frio
  note: los parametros que se incorporan en la s-function son: [nr thin tcin inter_name est]
      | con el parametro est establece si se parte del punto estacionario o no. De esta manera si est= 1 se parte del putno guardado (para cada intercambiador) de estado estacionario. Los mismos deben estar en un .mat
      | En cambio si es est=0 se parte de un perfil lineal  desde las temperaturas de entrada para la corriente caliente y fria (thin y tcin), una vez que se llega el estado estacionario se guardan los valores finales en un .mat
      | dela forma dynamic_inter_(inter_name).mat   es por ello que se envia el nombre del intercambiador.
      | Generalmente para la primera vez que se corre la red se una est=0 para que llegue al estado estacionario y una vez que se alcanzó se vuelve a correr con est= 1 para hacer análisis de control
  "op hot - bypass " : Inport
  H In : Inport  Port=2
  C in : Inport  Port=3
  "op cold - bypass " : Inport  Port=4
  Area : Step  Time=8  Before=aE2  After=aE2  SampleTime=0
  Fc : Fcn  Expr=u(2)
  Fh : Fcn  Expr=u(2)
  Mux : Mux
  Mux1 : Mux  Inputs=3
  Mux2 : Mux  Inputs=3
  Mux3 : Mux  Inputs=2
  Mux6 : Mux  Inputs=2
  S-Function2 : S-Function  FunctionName=Int_er  Parameters=10 443 323 111 2  SFunctionDeploymentMode=off  EnableBusSupport=off
  Saturation1 : Saturate  UpperLimit=1  LowerLimit=0
  Saturation2 : Saturate  UpperLimit=1  LowerLimit=0
  Scope1 : Scope
  Scope8 : Scope
  Tcin1 : Fcn  Expr=u(1)
  Tcin2 : Fcn  Expr=u(1)
  Tcout : Fcn  Expr=u(11)
  Tcout1 : Fcn  Expr=u(1)
  Tcout2 : Fcn  Expr=u(1)
  Thout : Fcn  Expr=u(10)
  To Workspace : ToWorkspace  VariableName=simout_int_E2  SampleTime=-1
  bypass : Subsystem
  bypass1 : Subsystem
  fac : Step  After=0  SampleTime=0
  hc : Fcn  Expr=u(3)
  hh : Fcn  Expr=u(3)
  mux : Subsystem
  mux1 : Subsystem
  valvula 1 : Subsystem
  valvula 2 : Subsystem
  H out : Outport  VectorParamsAs1DForOutWhenUnconnected=off
  C out : Outport  Port=2  VectorParamsAs1DForOutWhenUnconnected=off
  wires:
  Tcin2/1 -> Mux3/1
  Tcout2/1 -> Mux3/2
  Mux3/1 -> Scope1/1
  Tcin1/1 -> Mux6/2
  Tcout1/1 -> Mux6/1
  Mux6/1 -> Scope8/1
  bypass1/2(" 2") -> mux1/2(F2)
  bypass1/1(" 1") -> Mux/2, Fc/1, hc/1
  mux1/1("F ") -> C out/1, Tcout1/1
  Mux2/1 -> mux1/1(F1)
  mux/1("F ") -> H out/1, Tcout2/1
  "op cold - bypass "/1 -> valvula 2/1(In1)
  C in/1 -> bypass1/1(1), Tcin1/1
  "op hot - bypass "/1 -> valvula 1/1(In1)
  bypass/2(" 2") -> mux/1(F1)
  Mux1/1 -> mux/2(F2)
  bypass/1(" 1") -> hh/1, Fh/1, Mux/1
  H In/1 -> bypass/1(1), Tcin2/1
  Area/1 -> Mux/4
  hh/1 -> Mux1/3
  hc/1 -> Mux2/3
  fac/1 -> Mux/3
  Mux/1 -> S-Function2/1
  S-Function2/1 -> Tcout/1, To Workspace/1, Thout/1
  Fh/1 -> Mux1/2
  Fc/1 -> Mux2/2
  Thout/1 -> Mux1/1
  Tcout/1 -> Mux2/1
  Saturation1/1 -> bypass1/2(u122)
  Saturation2/1 -> bypass/2(u122)
  valvula 1/1(Out1) -> Saturation2/1
  valvula 2/1(Out1) -> Saturation1/1

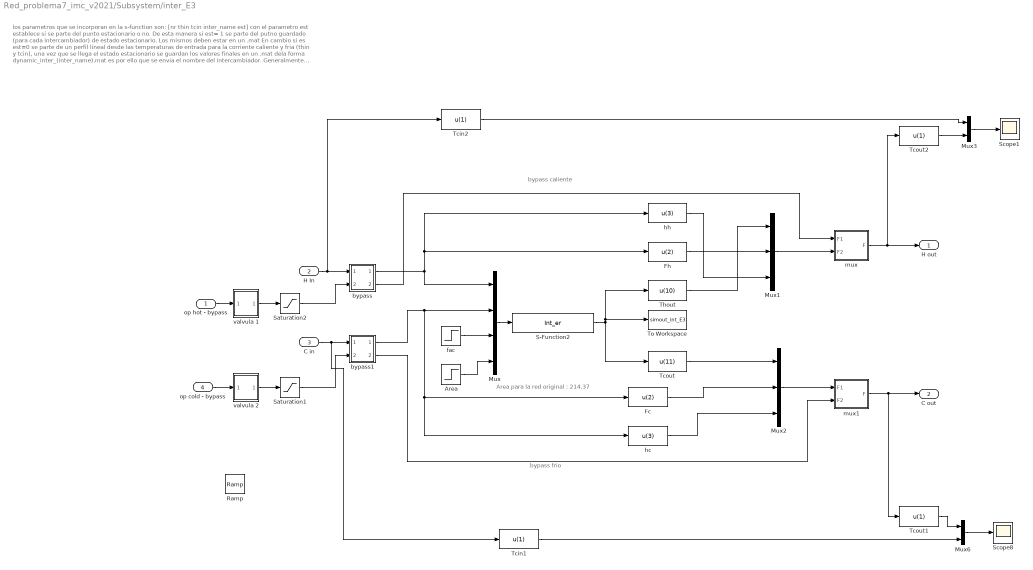
== system Red_problema7_imc_v2021/Subsystem/inter_E3 ==
  note: Area para la red original : 214.37
  note: bypass caliente
  note: bypass frio
  note: los parametros que se incorporan en la s-function son: [nr thin tcin inter_name est]
      | con el parametro est establece si se parte del punto estacionario o no. De esta manera si est= 1 se parte del putno guardado (para cada intercambiador) de estado estacionario. Los mismos deben estar en un .mat
      | En cambio si es est=0 se parte de un perfil lineal  desde las temperaturas de entrada para la corriente caliente y fria (thin y tcin), una vez que se llega el estado estacionario se guardan los valores finales en un .mat
      | dela forma dynamic_inter_(inter_name).mat   es por ello que se envia el nombre del intercambiador.
      | Generalmente para la primera vez que se corre la red se una est=0 para que llegue al estado estacionario y una vez que se alcanzó se vuelve a correr con est= 1 para hacer análisis de control
  "op hot - bypass " : Inport
  H In : Inport  Port=2
  C in : Inport  Port=3
  "op cold - bypass " : Inport  Port=4
  Area : Step  Time=8  Before=aE3  After=aE3  SampleTime=0
  Fc : Fcn  Expr=u(2)
  Fh : Fcn  Expr=u(2)
  Mux : Mux
  Mux1 : Mux  Inputs=3
  Mux2 : Mux  Inputs=3
  Mux3 : Mux  Inputs=2
  Mux6 : Mux  Inputs=2
  Ramp : simulink/Sources/Ramp  slope=1  start=0  InitialOutput=0
  S-Function2 : S-Function  FunctionName=Int_er  Parameters=10 493 433 222 2  SFunctionDeploymentMode=off  EnableBusSupport=off
  Saturation1 : Saturate  UpperLimit=1  LowerLimit=0
  Saturation2 : Saturate  UpperLimit=1  LowerLimit=0
  Scope1 : Scope
  Scope8 : Scope
  Tcin1 : Fcn  Expr=u(1)
  Tcin2 : Fcn  Expr=u(1)
  Tcout : Fcn  Expr=u(11)
  Tcout1 : Fcn  Expr=u(1)
  Tcout2 : Fcn  Expr=u(1)
  Thout : Fcn  Expr=u(10)
  To Workspace : ToWorkspace  VariableName=simout_int_E3  SampleTime=-1
  bypass : Subsystem
  bypass1 : Subsystem
  fac : Step  After=0  SampleTime=0
  hc : Fcn  Expr=u(3)
  hh : Fcn  Expr=u(3)
  mux : Subsystem
  mux1 : Subsystem
  valvula 1 : Subsystem
  valvula 2 : Subsystem
  H out : Outport  VectorParamsAs1DForOutWhenUnconnected=off
  C out : Outport  Port=2  VectorParamsAs1DForOutWhenUnconnected=off
  wires:
  Tcin2/1 -> Mux3/1
  Tcout2/1 -> Mux3/2
  Mux3/1 -> Scope1/1
  Tcin1/1 -> Mux6/2
  Tcout1/1 -> Mux6/1
  Mux6/1 -> Scope8/1
  bypass1/1(" 1") -> Mux/2, Fc/1, hc/1
  mux1/1("F ") -> C out/1, Tcout1/1
  Mux2/1 -> mux1/1(F1)
  mux/1("F ") -> H out/1, Tcout2/1
  "op cold - bypass "/1 -> valvula 2/1(In1)
  C in/1 -> bypass1/1(1), Tcin1/1
  "op hot - bypass "/1 -> valvula 1/1(In1)
  Mux1/1 -> mux/2(F2)
  bypass/1(" 1") -> hh/1, Fh/1, Mux/1
  H In/1 -> bypass/1(1), Tcin2/1
  Area/1 -> Mux/4
  hh/1 -> Mux1/3
  hc/1 -> Mux2/3
  fac/1 -> Mux/3
  Mux/1 -> S-Function2/1
  S-Function2/1 -> Tcout/1, To Workspace/1, Thout/1
  Fh/1 -> Mux1/2
  Fc/1 -> Mux2/2
  Thout/1 -> Mux1/1
  Tcout/1 -> Mux2/1
  Saturation1/1 -> bypass1/2(u122)
  Saturation2/1 -> bypass/2(u122)
  bypass/2(" 2") -> mux/1(F1)
  bypass1/2(" 2") -> mux1/2(F2)
  valvula 1/1(Out1) -> Saturation2/1
  valvula 2/1(Out1) -> Saturation1/1

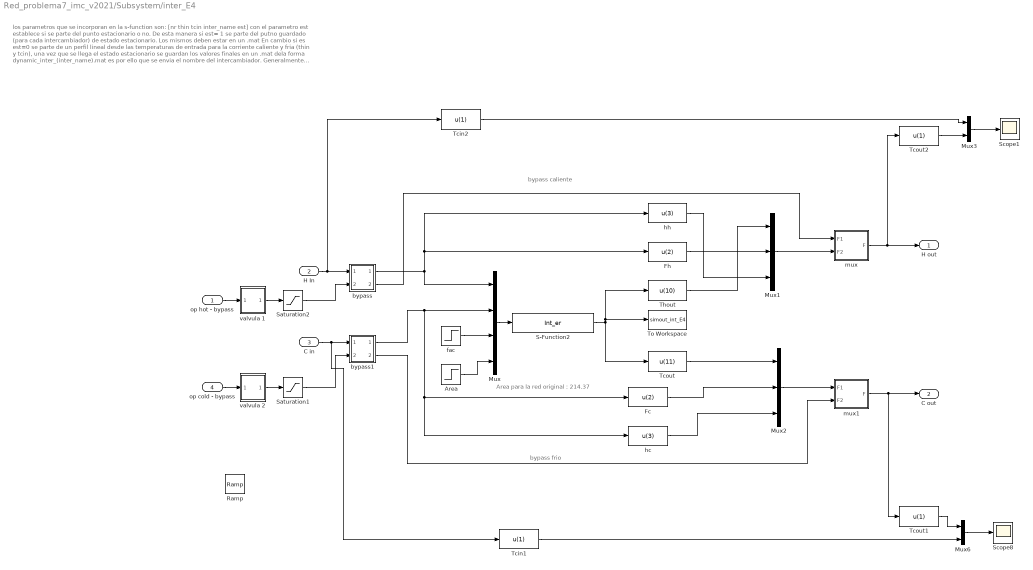
== system Red_problema7_imc_v2021/Subsystem/inter_E4 ==
  note: Area para la red original : 214.37
  note: bypass caliente
  note: bypass frio
  note: los parametros que se incorporan en la s-function son: [nr thin tcin inter_name est]
      | con el parametro est establece si se parte del punto estacionario o no. De esta manera si est= 1 se parte del putno guardado (para cada intercambiador) de estado estacionario. Los mismos deben estar en un .mat
      | En cambio si es est=0 se parte de un perfil lineal  desde las temperaturas de entrada para la corriente caliente y fria (thin y tcin), una vez que se llega el estado estacionario se guardan los valores finales en un .mat
      | dela forma dynamic_inter_(inter_name).mat   es por ello que se envia el nombre del intercambiador.
      | Generalmente para la primera vez que se corre la red se una est=0 para que llegue al estado estacionario y una vez que se alcanzó se vuelve a correr con est= 1 para hacer análisis de control
  "op hot - bypass " : Inport
  H In : Inport  Port=2
  C in : Inport  Port=3
  "op cold - bypass " : Inport  Port=4
  Area : Step  Time=8  Before=aE4  After=aE4  SampleTime=0
  Fc : Fcn  Expr=u(2)
  Fh : Fcn  Expr=u(2)
  Mux : Mux
  Mux1 : Mux  Inputs=3
  Mux2 : Mux  Inputs=3
  Mux3 : Mux  Inputs=2
  Mux6 : Mux  Inputs=2
  Ramp : simulink/Sources/Ramp  slope=1  start=0  InitialOutput=0
  S-Function2 : S-Function  FunctionName=Int_er  Parameters=10 443 343 213 2  SFunctionDeploymentMode=off  EnableBusSupport=off
  Saturation1 : Saturate  UpperLimit=1  LowerLimit=0
  Saturation2 : Saturate  UpperLimit=1  LowerLimit=0
  Scope1 : Scope
  Scope8 : Scope
  Tcin1 : Fcn  Expr=u(1)
  Tcin2 : Fcn  Expr=u(1)
  Tcout : Fcn  Expr=u(11)
  Tcout1 : Fcn  Expr=u(1)
  Tcout2 : Fcn  Expr=u(1)
  Thout : Fcn  Expr=u(10)
  To Workspace : ToWorkspace  VariableName=simout_int_E4  SampleTime=-1
  bypass : Subsystem
  bypass1 : Subsystem
  fac : Step  After=0  SampleTime=0
  hc : Fcn  Expr=u(3)
  hh : Fcn  Expr=u(3)
  mux : Subsystem
  mux1 : Subsystem
  valvula 1 : Subsystem
  valvula 2 : Subsystem
  H out : Outport  VectorParamsAs1DForOutWhenUnconnected=off
  C out : Outport  Port=2  VectorParamsAs1DForOutWhenUnconnected=off
  wires:
  Tcin2/1 -> Mux3/1
  Tcout2/1 -> Mux3/2
  Mux3/1 -> Scope1/1
  Tcin1/1 -> Mux6/2
  Tcout1/1 -> Mux6/1
  Mux6/1 -> Scope8/1
  bypass1/2(" 2") -> mux1/2(F2)
  bypass1/1(" 1") -> Mux/2, Fc/1, hc/1
  mux1/1("F ") -> C out/1, Tcout1/1
  Mux2/1 -> mux1/1(F1)
  mux/1("F ") -> H out/1, Tcout2/1
  "op cold - bypass "/1 -> valvula 2/1(In1)
  C in/1 -> bypass1/1(1), Tcin1/1
  "op hot - bypass "/1 -> valvula 1/1(In1)
  bypass/2(" 2") -> mux/1(F1)
  Mux1/1 -> mux/2(F2)
  bypass/1(" 1") -> hh/1, Fh/1, Mux/1
  H In/1 -> bypass/1(1), Tcin2/1
  Area/1 -> Mux/4
  hh/1 -> Mux1/3
  hc/1 -> Mux2/3
  fac/1 -> Mux/3
  Mux/1 -> S-Function2/1
  S-Function2/1 -> Tcout/1, To Workspace/1, Thout/1
  Fh/1 -> Mux1/2
  Fc/1 -> Mux2/2
  Thout/1 -> Mux1/1
  Tcout/1 -> Mux2/1
  Saturation1/1 -> bypass1/2(u122)
  Saturation2/1 -> bypass/2(u122)
  valvula 1/1(Out1) -> Saturation2/1
  valvula 2/1(Out1) -> Saturation1/1

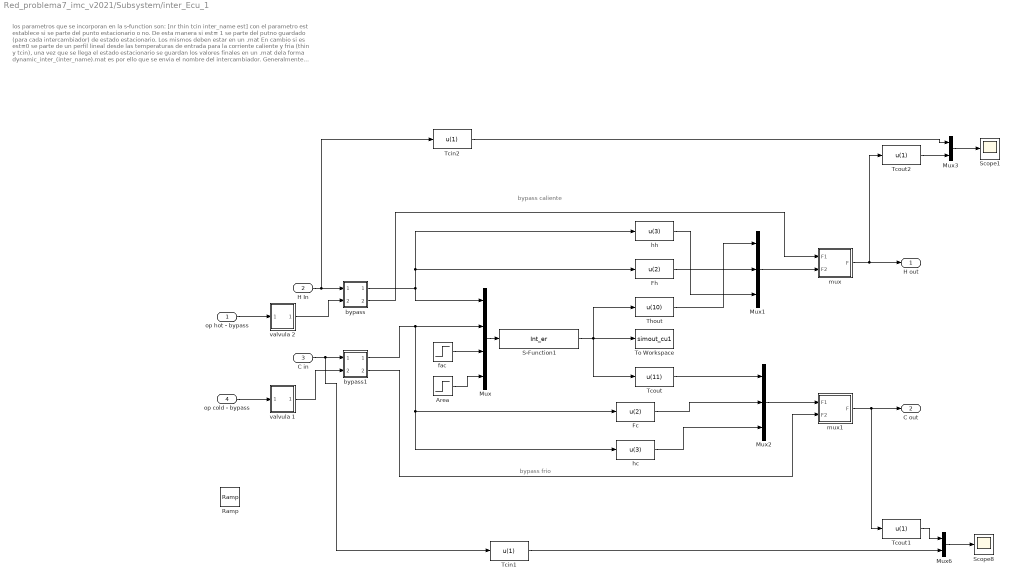
== system Red_problema7_imc_v2021/Subsystem/inter_Ecu_1 ==
  note: bypass caliente
  note: bypass frio
  note: los parametros que se incorporan en la s-function son: [nr thin tcin inter_name est]
      | con el parametro est establece si se parte del punto estacionario o no. De esta manera si est= 1 se parte del putno guardado (para cada intercambiador) de estado estacionario. Los mismos deben estar en un .mat
      | En cambio si es est=0 se parte de un perfil lineal  desde las temperaturas de entrada para la corriente caliente y fria (thin y tcin), una vez que se llega el estado estacionario se guardan los valores finales en un .mat
      | dela forma dynamic_inter_(inter_name).mat   es por ello que se envia el nombre del intercambiador.
      | Generalmente para la primera vez que se corre la red se una est=0 para que llegue al estado estacionario y una vez que se alcanzó se vuelve a correr con est= 1 para hacer análisis de control
  "op hot - bypass " : Inport
  H In : Inport  Port=2
  C in : Inport  Port=3
  "op cold - bypass " : Inport  Port=4
  Area : Step  Time=8  Before=aEcu1  After=aEcu1  SampleTime=0
  Fc : Fcn  Expr=u(2)
  Fh : Fcn  Expr=u(2)
  Mux : Mux
  Mux1 : Mux  Inputs=3
  Mux2 : Mux  Inputs=3
  Mux3 : Mux  Inputs=2
  Mux6 : Mux  Inputs=2
  Ramp : simulink/Sources/Ramp  slope=1  start=0  InitialOutput=0
  S-Function1 : S-Function  FunctionName=Int_er  Parameters=10 443 288 01 2  SFunctionDeploymentMode=off  EnableBusSupport=off
  Scope1 : Scope
  Scope8 : Scope
  Tcin1 : Fcn  Expr=u(1)
  Tcin2 : Fcn  Expr=u(1)
  Tcout : Fcn  Expr=u(11)
  Tcout1 : Fcn  Expr=u(1)
  Tcout2 : Fcn  Expr=u(1)
  Thout : Fcn  Expr=u(10)
  To Workspace : ToWorkspace  VariableName=simout_cu1  SampleTime=-1
  bypass : Subsystem
  bypass1 : Subsystem
  fac : Step  After=0  SampleTime=0
  hc : Fcn  Expr=u(3)
  hh : Fcn  Expr=u(3)
  mux : Subsystem
  mux1 : Subsystem
  valvula 1 : Subsystem
  valvula 2 : Subsystem
  H out : Outport  VectorParamsAs1DForOutWhenUnconnected=off
  C out : Outport  Port=2  VectorParamsAs1DForOutWhenUnconnected=off
  wires:
  Tcin2/1 -> Mux3/1
  Tcout2/1 -> Mux3/2
  Mux3/1 -> Scope1/1
  Tcin1/1 -> Mux6/2
  Tcout1/1 -> Mux6/1
  Mux6/1 -> Scope8/1
  bypass1/2(" 2") -> mux1/2(F2)
  bypass1/1(" 1") -> Mux/2, Fc/1, hc/1
  mux1/1("F ") -> C out/1, Tcout1/1
  Mux2/1 -> mux1/1(F1)
  mux/1("F ") -> H out/1, Tcout2/1
  "op cold - bypass "/1 -> valvula 1/1(In1)
  C in/1 -> bypass1/1(1), Tcin1/1
  "op hot - bypass "/1 -> valvula 2/1(In1)
  bypass/2(" 2") -> mux/1(F1)
  Mux1/1 -> mux/2(F2)
  bypass/1(" 1") -> hh/1, Fh/1, Mux/1
  H In/1 -> bypass/1(1), Tcin2/1
  Area/1 -> Mux/4
  hh/1 -> Mux1/3
  hc/1 -> Mux2/3
  fac/1 -> Mux/3
  Mux/1 -> S-Function1/1
  S-Function1/1 -> Thout/1, To Workspace/1, Tcout/1
  Fh/1 -> Mux1/2
  Fc/1 -> Mux2/2
  Thout/1 -> Mux1/1
  Tcout/1 -> Mux2/1
  valvula 1/1(Out1) -> bypass1/2(u122)
  valvula 2/1(Out1) -> bypass/2(u122)

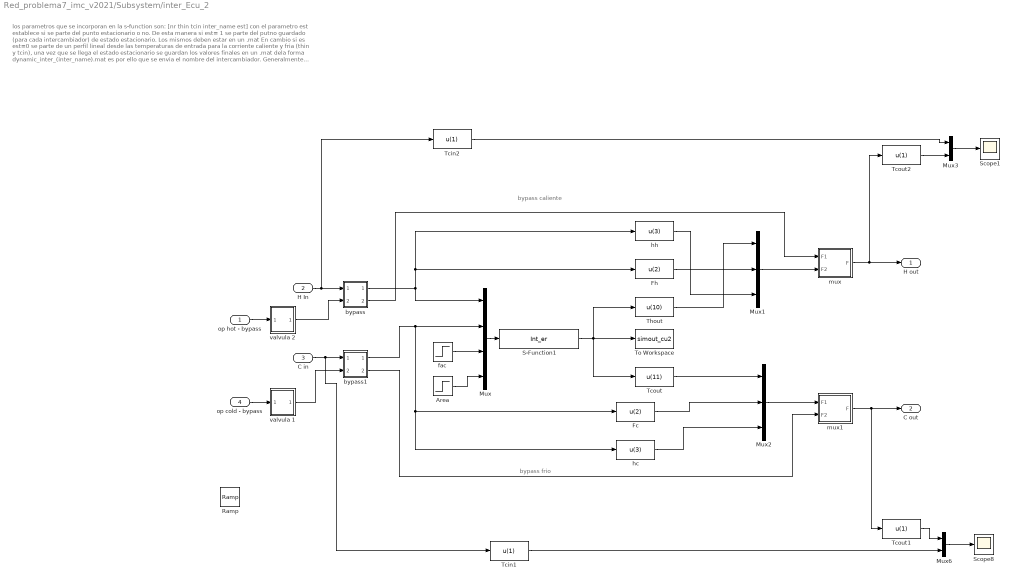
== system Red_problema7_imc_v2021/Subsystem/inter_Ecu_2 ==
  note: bypass caliente
  note: bypass frio
  note: los parametros que se incorporan en la s-function son: [nr thin tcin inter_name est]
      | con el parametro est establece si se parte del punto estacionario o no. De esta manera si est= 1 se parte del putno guardado (para cada intercambiador) de estado estacionario. Los mismos deben estar en un .mat
      | En cambio si es est=0 se parte de un perfil lineal  desde las temperaturas de entrada para la corriente caliente y fria (thin y tcin), una vez que se llega el estado estacionario se guardan los valores finales en un .mat
      | dela forma dynamic_inter_(inter_name).mat   es por ello que se envia el nombre del intercambiador.
      | Generalmente para la primera vez que se corre la red se una est=0 para que llegue al estado estacionario y una vez que se alcanzó se vuelve a correr con est= 1 para hacer análisis de control
  "op hot - bypass " : Inport
  H In : Inport  Port=2
  C in : Inport  Port=3
  "op cold - bypass " : Inport  Port=4
  Area : Step  Time=0  Before=aEcu2  After=aEcu2  SampleTime=0
  Fc : Fcn  Expr=u(2)
  Fh : Fcn  Expr=u(2)
  Mux : Mux
  Mux1 : Mux  Inputs=3
  Mux2 : Mux  Inputs=3
  Mux3 : Mux  Inputs=2
  Mux6 : Mux  Inputs=2
  Ramp : simulink/Sources/Ramp  slope=1  start=0  InitialOutput=0
  S-Function1 : S-Function  FunctionName=Int_er  Parameters=10 343 288 02 2  SFunctionDeploymentMode=off  EnableBusSupport=off
  Scope1 : Scope
  Scope8 : Scope
  Tcin1 : Fcn  Expr=u(1)
  Tcin2 : Fcn  Expr=u(1)
  Tcout : Fcn  Expr=u(11)
  Tcout1 : Fcn  Expr=u(1)
  Tcout2 : Fcn  Expr=u(1)
  Thout : Fcn  Expr=u(10)
  To Workspace : ToWorkspace  VariableName=simout_cu2  SampleTime=-1
  bypass : Subsystem
  bypass1 : Subsystem
  fac : Step  After=0  SampleTime=0
  hc : Fcn  Expr=u(3)
  hh : Fcn  Expr=u(3)
  mux : Subsystem
  mux1 : Subsystem
  valvula 1 : Subsystem
  valvula 2 : Subsystem
  H out : Outport  VectorParamsAs1DForOutWhenUnconnected=off
  C out : Outport  Port=2  VectorParamsAs1DForOutWhenUnconnected=off
  wires:
  Tcin2/1 -> Mux3/1
  Tcout2/1 -> Mux3/2
  Mux3/1 -> Scope1/1
  Tcin1/1 -> Mux6/2
  Tcout1/1 -> Mux6/1
  Mux6/1 -> Scope8/1
  bypass1/2(" 2") -> mux1/2(F2)
  bypass1/1(" 1") -> Mux/2, Fc/1, hc/1
  mux1/1("F ") -> C out/1, Tcout1/1
  Mux2/1 -> mux1/1(F1)
  mux/1("F ") -> H out/1, Tcout2/1
  "op cold - bypass "/1 -> valvula 1/1(In1)
  C in/1 -> bypass1/1(1), Tcin1/1
  "op hot - bypass "/1 -> valvula 2/1(In1)
  bypass/2(" 2") -> mux/1(F1)
  Mux1/1 -> mux/2(F2)
  bypass/1(" 1") -> hh/1, Fh/1, Mux/1
  H In/1 -> bypass/1(1), Tcin2/1
  Area/1 -> Mux/4
  hh/1 -> Mux1/3
  hc/1 -> Mux2/3
  fac/1 -> Mux/3
  Mux/1 -> S-Function1/1
  S-Function1/1 -> Thout/1, To Workspace/1, Tcout/1
  Fh/1 -> Mux1/2
  Fc/1 -> Mux2/2
  Thout/1 -> Mux1/1
  Tcout/1 -> Mux2/1
  valvula 1/1(Out1) -> bypass1/2(u122)
  valvula 2/1(Out1) -> bypass/2(u122)

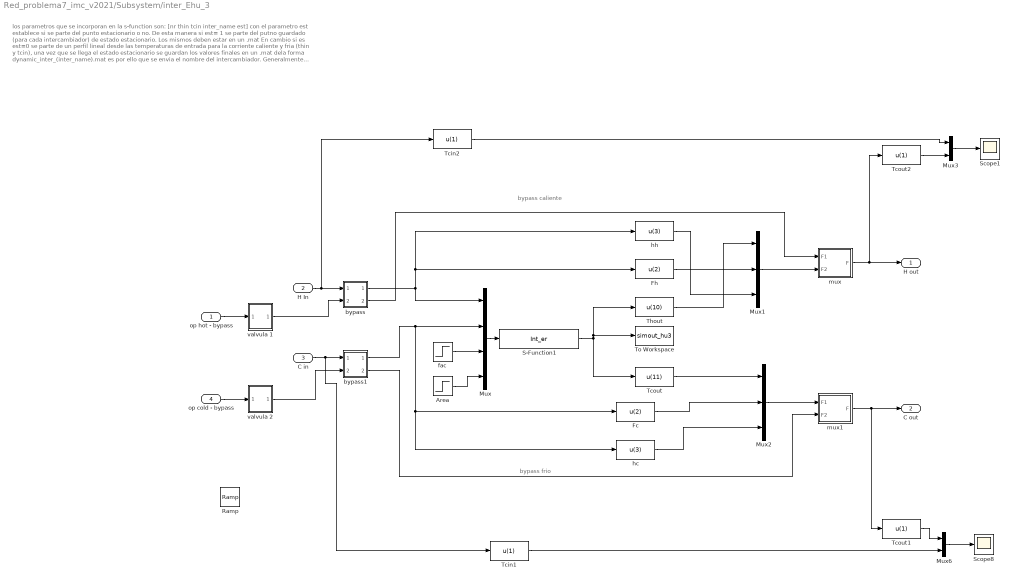
== system Red_problema7_imc_v2021/Subsystem/inter_Ehu_3 ==
  note: bypass caliente
  note: bypass frio
  note: los parametros que se incorporan en la s-function son: [nr thin tcin inter_name est]
      | con el parametro est establece si se parte del punto estacionario o no. De esta manera si est= 1 se parte del putno guardado (para cada intercambiador) de estado estacionario. Los mismos deben estar en un .mat
      | En cambio si es est=0 se parte de un perfil lineal  desde las temperaturas de entrada para la corriente caliente y fria (thin y tcin), una vez que se llega el estado estacionario se guardan los valores finales en un .mat
      | dela forma dynamic_inter_(inter_name).mat   es por ello que se envia el nombre del intercambiador.
      | Generalmente para la primera vez que se corre la red se una est=0 para que llegue al estado estacionario y una vez que se alcanzó se vuelve a correr con est= 1 para hacer análisis de control
  "op hot - bypass " : Inport
  H In : Inport  Port=2
  C in : Inport  Port=3
  "op cold - bypass " : Inport  Port=4
  Area : Step  Time=8  Before=aEhu2  After=aEhu2  SampleTime=0
  Fc : Fcn  Expr=u(2)
  Fh : Fcn  Expr=u(2)
  Mux : Mux
  Mux1 : Mux  Inputs=3
  Mux2 : Mux  Inputs=3
  Mux3 : Mux  Inputs=2
  Mux6 : Mux  Inputs=2
  Ramp : simulink/Sources/Ramp  slope=1  start=0  InitialOutput=0
  S-Function1 : S-Function  FunctionName=Int_er  Parameters=10 523 471 03 2  SFunctionDeploymentMode=off  EnableBusSupport=off
  Scope1 : Scope
  Scope8 : Scope
  Tcin1 : Fcn  Expr=u(1)
  Tcin2 : Fcn  Expr=u(1)
  Tcout : Fcn  Expr=u(11)
  Tcout1 : Fcn  Expr=u(1)
  Tcout2 : Fcn  Expr=u(1)
  Thout : Fcn  Expr=u(10)
  To Workspace : ToWorkspace  VariableName=simout_hu3  SampleTime=-1
  bypass : Subsystem
  bypass1 : Subsystem
  fac : Step  After=0  SampleTime=0
  hc : Fcn  Expr=u(3)
  hh : Fcn  Expr=u(3)
  mux : Subsystem
  mux1 : Subsystem
  valvula 1 : Subsystem
  valvula 2 : Subsystem
  H out : Outport  VectorParamsAs1DForOutWhenUnconnected=off
  C out : Outport  Port=2  VectorParamsAs1DForOutWhenUnconnected=off
  wires:
  Tcin2/1 -> Mux3/1
  Tcout2/1 -> Mux3/2
  Mux3/1 -> Scope1/1
  Tcin1/1 -> Mux6/2
  Tcout1/1 -> Mux6/1
  Mux6/1 -> Scope8/1
  bypass1/2(" 2") -> mux1/2(F2)
  bypass1/1(" 1") -> Mux/2, Fc/1, hc/1
  mux1/1("F ") -> C out/1, Tcout1/1
  Mux2/1 -> mux1/1(F1)
  mux/1("F ") -> H out/1, Tcout2/1
  "op cold - bypass "/1 -> valvula 2/1(In1)
  C in/1 -> bypass1/1(1), Tcin1/1
  "op hot - bypass "/1 -> valvula 1/1(In1)
  bypass/2(" 2") -> mux/1(F1)
  Mux1/1 -> mux/2(F2)
  bypass/1(" 1") -> hh/1, Fh/1, Mux/1
  H In/1 -> bypass/1(1), Tcin2/1
  Area/1 -> Mux/4
  hh/1 -> Mux1/3
  hc/1 -> Mux2/3
  fac/1 -> Mux/3
  Mux/1 -> S-Function1/1
  S-Function1/1 -> Tcout/1, To Workspace/1, Thout/1
  Fh/1 -> Mux1/2
  Fc/1 -> Mux2/2
  Thout/1 -> Mux1/1
  Tcout/1 -> Mux2/1
  valvula 1/1(Out1) -> bypass/2(u122)
  valvula 2/1(Out1) -> bypass1/2(u122)

== system Red_problema7_imc_v2021/Subsystem/Corriente C1/valvula 3 ==
  In1 : Inport
  Gain : Gain  Gain=s1
  Gain1 : Gain  Gain=s1
  Integrator : Integrator  InitialCondition=[Thuin fhu2 hhu]
  Sum : Sum  Inputs=|+-
  Out1 : Outport  VectorParamsAs1DForOutWhenUnconnected=off
  wires:
  Gain1/1 -> Sum/2
  Integrator/1 -> Out1/1, Gain1/1
  Sum/1 -> Integrator/1
  Gain/1 -> Sum/1
  In1/1 -> Gain/1

== system Red_problema7_imc_v2021/Subsystem/Corriente C2/valvula 3 ==
  In1 : Inport
  Gain : Gain  Gain=s1
  Gain1 : Gain  Gain=s1
  Integrator : Integrator  InitialCondition=[Thuin fhu2 hhu]
  Sum : Sum  Inputs=|+-
  Out1 : Outport  VectorParamsAs1DForOutWhenUnconnected=off
  wires:
  Gain1/1 -> Sum/2
  Integrator/1 -> Out1/1, Gain1/1
  Sum/1 -> Integrator/1
  Gain/1 -> Sum/1
  In1/1 -> Gain/1

== system Red_problema7_imc_v2021/Subsystem/Corriente H1/valvula 3 ==
  In1 : Inport
  Gain : Gain  Gain=s1
  Gain1 : Gain  Gain=s1
  Integrator : Integrator  InitialCondition=[Thuin fhu2 hhu]
  Sum : Sum  Inputs=|+-
  Out1 : Outport  VectorParamsAs1DForOutWhenUnconnected=off
  wires:
  Gain1/1 -> Sum/2
  Integrator/1 -> Out1/1, Gain1/1
  Sum/1 -> Integrator/1
  Gain/1 -> Sum/1
  In1/1 -> Gain/1

== system Red_problema7_imc_v2021/Subsystem/Corriente H2/valvula 3 ==
  In1 : Inport
  Gain : Gain  Gain=s1
  Gain1 : Gain  Gain=s1
  Integrator : Integrator  InitialCondition=[Thuin fhu2 hhu]
  Sum : Sum  Inputs=|+-
  Out1 : Outport  VectorParamsAs1DForOutWhenUnconnected=off
  wires:
  Gain1/1 -> Sum/2
  Integrator/1 -> Out1/1, Gain1/1
  Sum/1 -> Integrator/1
  Gain/1 -> Sum/1
  In1/1 -> Gain/1
